simulink model "trifasikos_ask53_trifasikos"  (R2021a)
settings: Solver=ode23tb  StartTime=0.0  StopTime=5.2  MaxStep=1e-4  RelTol=1e-3
libraries: spsSaturableTransformerLib x6, spsCurrentMeasurementLib x5, spsVoltageMeasurementLib x5, spsNeutralLib x4, spsSeriesRLCBranchLib x4, spsControlledVoltageSourceLib x3, spsRMSLib x3, simulink x1, spsMeanLib x1, spsPower3phInstantaneousLib x1, spsDCVoltageSourceLib x1, spspowerguiLib x1
settings Model: Creator=User  LastModifiedBy=epape
settings SolverCC: AlgebraicLoopSolver=TrustRegion
settings DebuggingCC: SFMachineParentedDataDiag=warning

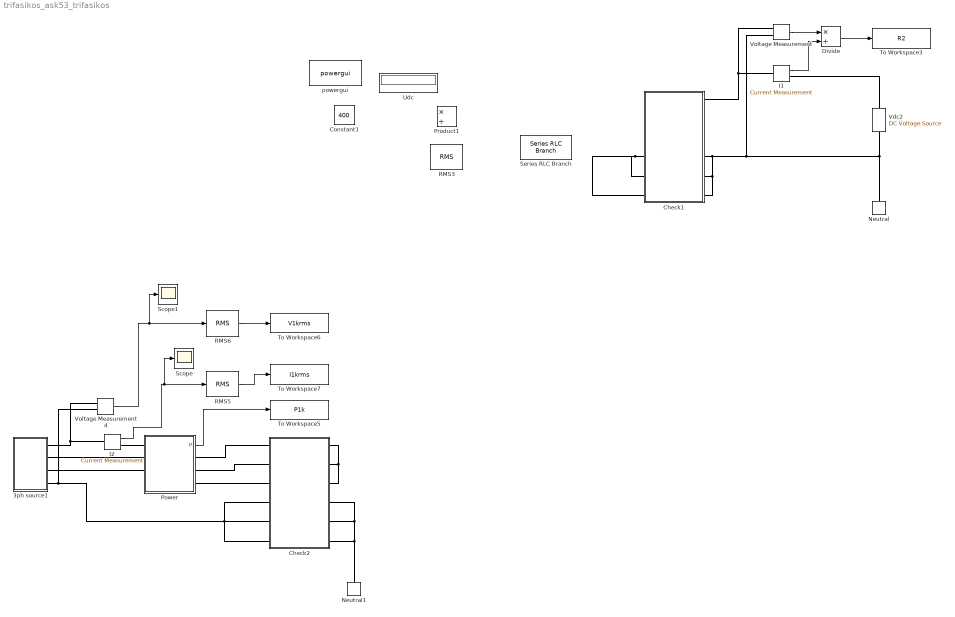
== system trifasikos_ask53_trifasikos ==
  3ph source1 : Subsystem  mask{Vrms=400}
      mask prompts: Vrms "VLL,rms (V)"
  Check1 : Subsystem  mask{PN=12, U1N=230, U2N=115}
      mask prompts: PN "PN (kVA)"; U1N "U1Nph (V)"; U2N "U2Nph (V)"
  Check2 : Subsystem  mask{PN=12, U1N=230, U2N=115}
      mask prompts: PN "PN (kVA)"; U1N "U1Nph (V)"; U2N "U2Nph (V)"
  Constant1 : Constant  Value=400
  Divide : Product  Inputs=*/
  I1 : spsCurrentMeasurementLib/Current Measurement  PhasorSimulation=off  OutputType=Complex  PSBequivalent=0
  I2 : spsCurrentMeasurementLib/Current Measurement  PhasorSimulation=off  OutputType=Complex  PSBequivalent=0
  Neutral : spsNeutralLib/Neutral  LConnTagsString=a  NodeNumber=10
      settings: AttributesFormatString=node %<NodeNumber>  SourceProductBaseCode=PS
  Neutral1 : spsNeutralLib/Neutral  LConnTagsString=a  NodeNumber=10
      settings: AttributesFormatString=node %<NodeNumber>  SourceProductBaseCode=PS
  Power : Subsystem
      mask DialogControl Control2 Prompt: Three phase power measurement
  Product1 : Product  Inputs=*/
  RMS3 : spsRMSLib/RMS  TrueRMS=on  Freq=50  RMSInit=0  Ts=0
  RMS5 : spsRMSLib/RMS  TrueRMS=on  Freq=50  RMSInit=0  Ts=0
  RMS6 : spsRMSLib/RMS  TrueRMS=on  Freq=50  RMSInit=0  Ts=0
  Scope : Scope
  Scope1 : Scope
  Series RLC Branch : spsSeriesRLCBranchLib/Series RLC Branch  LConnTagsString=__new0  RConnTagsString=__new0  BranchType=RLC  Resistance=1  Inductance=1e-3  SetiL0=off  InitialCurrent=0  Capacitance=1e-6  Setx0=off  InitialVoltage=0  Measurements=None
  To Workspace3 : ToWorkspace  VariableName=R2  SaveFormat=Timeseries  SampleTime=-1
  To Workspace5 : ToWorkspace  VariableName=P1k  SaveFormat=Timeseries  SampleTime=-1
  To Workspace6 : ToWorkspace  VariableName=V1krms  SaveFormat=Timeseries  SampleTime=-1
  To Workspace7 : ToWorkspace  VariableName=I1krms  SaveFormat=Timeseries  SampleTime=-1
  Udc : Display
  Vdc2 : spsDCVoltageSourceLib/DC Voltage Source  Amplitude=10  Measurements=None
  Voltage Measurement : spsVoltageMeasurementLib/Voltage Measurement  PhasorSimulation=off  OutputType=Complex  PSBequivalent=0
  Voltage Measurement4 : spsVoltageMeasurementLib/Voltage Measurement  PhasorSimulation=off  OutputType=Complex  PSBequivalent=0
  powergui : spspowerguiLib/powergui  Priority=1  SimulationMode=Continuous  SampleTime=50e-6  frequency=60  Iterations=50  frequencyindice=50  Pbase=100e6  ErrMax=1e-4  UnitsV=kV  UnitsW=MW  buscounter=0  FunctionMessages=off  echomessages=off  EnableUseOfTLC=off  CurrentSourceSwitches=off  DisableSnubberDevices=off  DisableRonSwitches=off  DisableVfSwitches=off  DisplayEquations=off  AutomaticDiscreteSolvers=off  SolverType=Tustin/Backward Euler (TBE)  Interpol=off  ExternalGateDelay=off  methode=off  Ts=100  x0status=blocks  SPID=on  SwTol=0  HookPort=off  NonlinearTolerance=1e-4  nMaxIteration=100  ContinueOnMaxIteration=off  RestoreLinks=warning  ResistiveCurrentMeasurement=off  Frange=[0:2:500]  Ylog=off  Xlog=on  ShowGrid=off  save=off  variable=ZData  structure=0  ZoomFFT=off  StartTime=0.0  cycles=1  DisplayStyle=1  fundamental=60  FreqAxis=off  MaxFrequency=1000  frequencyindicesteady=1  RmsSteady=1  display=off
  wires:
  Divide/1 -> To Workspace3/1
  Voltage Measurement/1 -> Divide/1
  I1/1 -> Divide/2
  Power/1(P) -> To Workspace5/1
  RMS6/1 -> To Workspace6/1
  RMS5/1 -> To Workspace7/1
  Voltage Measurement4/1 -> Scope1/1, RMS6/1
  I2/1 -> Scope/1, RMS5/1
  connections:
  Check1/LConn4 -- Check1/LConn6 -- Check1/LConn5
  3ph source1/RConn4 -- Check2/LConn4 -- Check2/LConn6 -- Check2/LConn5 -- Voltage Measurement4/LConn2
  Neutral1/LConn1 -- Check2/RConn6 -- Check2/RConn4 -- Check2/RConn5
  Check1/RConn4 -- Voltage Measurement/LConn2 -- Neutral/LConn1 -- Vdc2/LConn1 -- Check1/RConn6 -- Check1/RConn5
  I1/LConn1 -- Check1/RConn1 -- Voltage Measurement/LConn1
  I1/RConn1 -- Vdc2/RConn1
  Power/RConn1 -- Check2/LConn1
  Power/RConn2 -- Check2/LConn2
  Power/RConn3 -- Check2/LConn3
  Voltage Measurement4/LConn1 -- 3ph source1/RConn1 -- I2/LConn1
  Power/LConn2 -- 3ph source1/RConn2
  Power/LConn3 -- 3ph source1/RConn3
  Power/LConn1 -- I2/RConn1
  Check2/RConn1 -- Check2/RConn3 -- Check2/RConn2

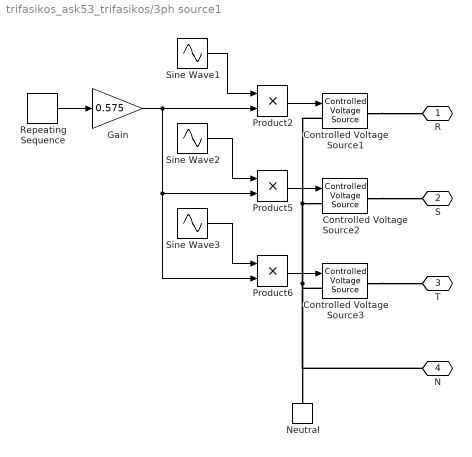
== system trifasikos_ask53_trifasikos/3ph source1 ==
  Controlled Voltage Source1 : spsControlledVoltageSourceLib/Controlled Voltage Source  Initialize=on  Source_Type=AC  Amplitude=0  Phase=0  Frequency=50  Measurements=Voltage
  Controlled Voltage Source2 : spsControlledVoltageSourceLib/Controlled Voltage Source  Initialize=on  Source_Type=AC  Amplitude=0  Phase=0  Frequency=50  Measurements=Voltage
  Controlled Voltage Source3 : spsControlledVoltageSourceLib/Controlled Voltage Source  Initialize=on  Source_Type=AC  Amplitude=0  Phase=0  Frequency=50  Measurements=Voltage
  Gain : Gain  Gain=0.575
  Neutral : spsNeutralLib/Neutral  LConnTagsString=a  NodeNumber=10
      settings: AttributesFormatString=node %<NodeNumber>  SourceProductBaseCode=PS
  Product2 : Product
  Product5 : Product
  Product6 : Product
  Repeating Sequence : simulink/Sources/Repeating Sequence  rep_seq_t=t  rep_seq_y=Vs
  Sine Wave1 : Sin  Amplitude=sqrt(2)  Frequency=100*pi  SampleTime=0
  Sine Wave2 : Sin  Amplitude=sqrt(2)  Frequency=100*pi  Phase=-2*pi/3  SampleTime=0
  Sine Wave3 : Sin  Amplitude=sqrt(2)  Frequency=100*pi  Phase=2*pi/3  SampleTime=0
  R : PMIOPort  Side=Right
  S : PMIOPort  Port=2  Side=Right
  T : PMIOPort  Port=3  Side=Right
  N : PMIOPort  Port=4  Side=Right
  wires:
  Repeating Sequence/1 -> Gain/1
  Product5/1 -> Controlled Voltage Source2/1
  Sine Wave2/1 -> Product5/1
  Product6/1 -> Controlled Voltage Source3/1
  Sine Wave3/1 -> Product6/1
  Product2/1 -> Controlled Voltage Source1/1
  Sine Wave1/1 -> Product2/1
  Gain/1 -> Product6/2, Product5/2, Product2/2
  connections:
  Controlled Voltage Source2/RConn1 -- S/RConn1
  Controlled Voltage Source1/LConn1 -- Controlled Voltage Source2/LConn1 -- Controlled Voltage Source3/LConn1 -- N/RConn1 -- Neutral/LConn1
  Controlled Voltage Source3/RConn1 -- T/RConn1
  Controlled Voltage Source1/RConn1 -- R/RConn1

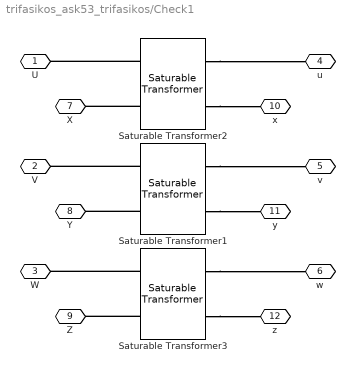
== system trifasikos_ask53_trifasikos/Check1 ==
  Saturable Transformer1 : spsSaturableTransformerLib/Saturable Transformer  ThreeWindings=off  Hysteresis=off  DataFile='hysteresis.mat'  Measurements=None  UNITS=pu  NominalPower=[4e3 50]  Winding1=[230 0.022273 0.015903]  Winding2=[122 0.024298 0.019083]  Winding3=[3.15e+05 0.00245 0.098001]  Saturation=[0 0;0.031714 0.76205;0.037813 0.86926;0.045538 0.94653;0.060175 1.0141;0.080911 1.0624;0.14637 1.159]  CoreLoss=35.539  BreakLoop=off  DiscreteSolver=Trapezoidal iterative  DataType=off  InitialFlux=0  TransfoNumber=1
      settings: SourceProductBaseCode=PS
  Saturable Transformer2 : spsSaturableTransformerLib/Saturable Transformer  ThreeWindings=off  Hysteresis=off  DataFile='hysteresis.mat'  Measurements=None  UNITS=SI  NominalPower=[4e3 50]  Winding1=[230 0.29456 0.00066946]  Winding2=[122 0.090413 0.00022602]  Winding3=[3.15e+05 60775 7738.2]  Saturation=[0 0;0.78001 0.789;0.93001 0.9;1.12 0.98;1.48 1.05;1.99 1.1;3.6 1.2]  CoreLoss=470  BreakLoop=off  DiscreteSolver=Trapezoidal iterative  DataType=on  InitialFlux=0  TransfoNumber=1
      settings: SourceProductBaseCode=PS
  Saturable Transformer3 : spsSaturableTransformerLib/Saturable Transformer  ThreeWindings=off  Hysteresis=off  DataFile='hysteresis.mat'  Measurements=None  UNITS=pu  NominalPower=[4e3 50]  Winding1=[230 0.022273 0.015903]  Winding2=[122 0.024298 0.019083]  Winding3=[3.15e+05 0.00245 0.098001]  Saturation=[0 0;0.031714 0.76205;0.037813 0.86926;0.045538 0.94653;0.060175 1.0141;0.080911 1.0624;0.14637 1.159]  CoreLoss=35.539  BreakLoop=off  DiscreteSolver=Trapezoidal iterative  DataType=off  InitialFlux=0  TransfoNumber=1
      settings: SourceProductBaseCode=PS
  U : PMIOPort  Side=Left
  V : PMIOPort  Port=2  Side=Left
  W : PMIOPort  Port=3  Side=Left
  u : PMIOPort  Port=4  Side=Right
  v : PMIOPort  Port=5  Side=Right
  w : PMIOPort  Port=6  Side=Right
  X : PMIOPort  Port=7  Side=Left
  Y : PMIOPort  Port=8  Side=Left
  Z : PMIOPort  Port=9  Side=Left
  x : PMIOPort  Port=10  Side=Right
  y : PMIOPort  Port=11  Side=Right
  z : PMIOPort  Port=12  Side=Right
  connections:
  Saturable Transformer1/LConn2 -- Y/RConn1
  Saturable Transformer2/LConn1 -- U/RConn1
  Saturable Transformer1/LConn1 -- V/RConn1
  Saturable Transformer3/LConn1 -- W/RConn1
  Saturable Transformer2/LConn2 -- X/RConn1
  Saturable Transformer3/LConn2 -- Z/RConn1
  Saturable Transformer2/RConn1 -- u/RConn1
  Saturable Transformer2/RConn2 -- x/RConn1
  Saturable Transformer1/RConn1 -- v/RConn1
  Saturable Transformer1/RConn2 -- y/RConn1
  Saturable Transformer3/RConn1 -- w/RConn1
  Saturable Transformer3/RConn2 -- z/RConn1

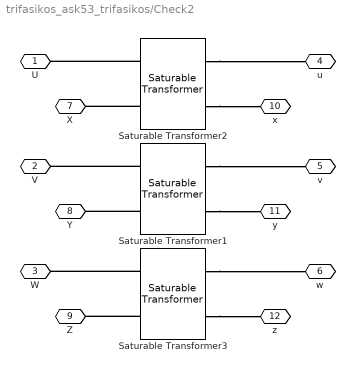
== system trifasikos_ask53_trifasikos/Check2 ==
  Saturable Transformer1 : spsSaturableTransformerLib/Saturable Transformer  ThreeWindings=off  Hysteresis=off  DataFile='hysteresis.mat'  Measurements=None  UNITS=pu  NominalPower=[4e3 50]  Winding1=[230 0.022273 0.015903]  Winding2=[122 0.024298 0.019083]  Winding3=[3.15e+05 0.00245 0.098001]  Saturation=[0 0;0.031714 0.76205;0.037813 0.86926;0.045538 0.94653;0.060175 1.0141;0.080911 1.0624;0.14637 1.159]  CoreLoss=35.539  BreakLoop=off  DiscreteSolver=Trapezoidal iterative  DataType=off  InitialFlux=0  TransfoNumber=1
      settings: SourceProductBaseCode=PS
  Saturable Transformer2 : spsSaturableTransformerLib/Saturable Transformer  ThreeWindings=off  Hysteresis=off  DataFile='hysteresis.mat'  Measurements=None  UNITS=SI  NominalPower=[4e3 50]  Winding1=[230 0.29456 0.00066946]  Winding2=[122 0.090413 0.00022602]  Winding3=[3.15e+05 60775 7738.2]  Saturation=[0 0;0.78001 0.789;0.93001 0.9;1.12 0.98;1.48 1.05;1.99 1.1;3.6 1.2]  CoreLoss=470  BreakLoop=off  DiscreteSolver=Trapezoidal iterative  DataType=on  InitialFlux=0  TransfoNumber=1
      settings: SourceProductBaseCode=PS
  Saturable Transformer3 : spsSaturableTransformerLib/Saturable Transformer  ThreeWindings=off  Hysteresis=off  DataFile='hysteresis.mat'  Measurements=None  UNITS=pu  NominalPower=[4e3 50]  Winding1=[230 0.022273 0.015903]  Winding2=[122 0.024298 0.019083]  Winding3=[3.15e+05 0.00245 0.098001]  Saturation=[0 0;0.031714 0.76205;0.037813 0.86926;0.045538 0.94653;0.060175 1.0141;0.080911 1.0624;0.14637 1.159]  CoreLoss=35.539  BreakLoop=off  DiscreteSolver=Trapezoidal iterative  DataType=off  InitialFlux=0  TransfoNumber=1
      settings: SourceProductBaseCode=PS
  U : PMIOPort  Side=Left
  V : PMIOPort  Port=2  Side=Left
  W : PMIOPort  Port=3  Side=Left
  u : PMIOPort  Port=4  Side=Right
  v : PMIOPort  Port=5  Side=Right
  w : PMIOPort  Port=6  Side=Right
  X : PMIOPort  Port=7  Side=Left
  Y : PMIOPort  Port=8  Side=Left
  Z : PMIOPort  Port=9  Side=Left
  x : PMIOPort  Port=10  Side=Right
  y : PMIOPort  Port=11  Side=Right
  z : PMIOPort  Port=12  Side=Right
  connections:
  Saturable Transformer1/LConn2 -- Y/RConn1
  Saturable Transformer2/LConn1 -- U/RConn1
  Saturable Transformer1/LConn1 -- V/RConn1
  Saturable Transformer3/LConn1 -- W/RConn1
  Saturable Transformer2/LConn2 -- X/RConn1
  Saturable Transformer3/LConn2 -- Z/RConn1
  Saturable Transformer2/RConn1 -- u/RConn1
  Saturable Transformer2/RConn2 -- x/RConn1
  Saturable Transformer1/RConn1 -- v/RConn1
  Saturable Transformer1/RConn2 -- y/RConn1
  Saturable Transformer3/RConn1 -- w/RConn1
  Saturable Transformer3/RConn2 -- z/RConn1

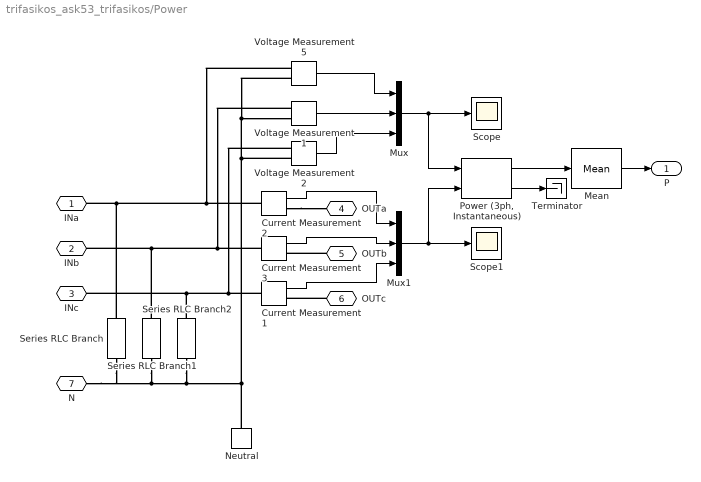
== system trifasikos_ask53_trifasikos/Power ==
  Current Measurement1 : spsCurrentMeasurementLib/Current Measurement  PhasorSimulation=off  OutputType=Complex  PSBequivalent=0
  Current Measurement2 : spsCurrentMeasurementLib/Current Measurement  PhasorSimulation=off  OutputType=Complex  PSBequivalent=0
  Current Measurement3 : spsCurrentMeasurementLib/Current Measurement  PhasorSimulation=off  OutputType=Complex  PSBequivalent=0
  Mean : spsMeanLib/Mean  Freq=50  Vinit=0  Ts=0
  Mux : Mux  Inputs=3
  Mux1 : Mux  Inputs=3
  Neutral : spsNeutralLib/Neutral  LConnTagsString=a  NodeNumber=10
      settings: AttributesFormatString=node %<NodeNumber>  SourceProductBaseCode=PS
  "Power (3ph, Instantaneous)" : spsPower3phInstantaneousLib/Power (3ph, Instantaneous)
  Scope : Scope
  Scope1 : Scope
  Series RLC Branch : spsSeriesRLCBranchLib/Series RLC Branch  LConnTagsString=__new0  RConnTagsString=__new0  BranchType=R  Resistance=1e6  Inductance=1e-3  SetiL0=off  InitialCurrent=0  Capacitance=1e-6  Setx0=off  InitialVoltage=0  Measurements=None
  Series RLC Branch1 : spsSeriesRLCBranchLib/Series RLC Branch  LConnTagsString=__new0  RConnTagsString=__new0  BranchType=R  Resistance=1e6  Inductance=1e-3  SetiL0=off  InitialCurrent=0  Capacitance=1e-6  Setx0=off  InitialVoltage=0  Measurements=None
  Series RLC Branch2 : spsSeriesRLCBranchLib/Series RLC Branch  LConnTagsString=__new0  RConnTagsString=__new0  BranchType=R  Resistance=1e6  Inductance=1e-3  SetiL0=off  InitialCurrent=0  Capacitance=1e-6  Setx0=off  InitialVoltage=0  Measurements=None
  Terminator : Terminator
  Voltage Measurement1 : spsVoltageMeasurementLib/Voltage Measurement  PhasorSimulation=off  OutputType=Complex  PSBequivalent=0
  Voltage Measurement2 : spsVoltageMeasurementLib/Voltage Measurement  PhasorSimulation=off  OutputType=Complex  PSBequivalent=0
  Voltage Measurement5 : spsVoltageMeasurementLib/Voltage Measurement  PhasorSimulation=off  OutputType=Complex  PSBequivalent=0
  INa : PMIOPort  Side=Left
  INb : PMIOPort  Port=2  Side=Left
  INc : PMIOPort  Port=3  Side=Left
  OUTa : PMIOPort  Port=4  Side=Right
  OUTb : PMIOPort  Port=5  Side=Right
  OUTc : PMIOPort  Port=6  Side=Right
  N : PMIOPort  Port=7  Side=Left
  P : Outport
  wires:
  "Power (3ph, Instantaneous)"/1 -> Mean/1
  Mux/1 -> "Power (3ph, Instantaneous)"/1, Scope/1
  Voltage Measurement5/1 -> Mux/1
  Mux1/1 -> "Power (3ph, Instantaneous)"/2, Scope1/1
  Voltage Measurement1/1 -> Mux/2
  Voltage Measurement2/1 -> Mux/3
  Current Measurement3/1 -> Mux1/2
  Current Measurement2/1 -> Mux1/1
  Current Measurement1/1 -> Mux1/3
  "Power (3ph, Instantaneous)"/2 -> Terminator/1
  Mean/1 -> P/1
  connections:
  Current Measurement1/LConn1 -- Voltage Measurement2/LConn1 -- Series RLC Branch2/LConn1 -- INc/RConn1
  Current Measurement3/LConn1 -- Voltage Measurement1/LConn1 -- Series RLC Branch1/LConn1 -- INb/RConn1
  Current Measurement2/LConn1 -- Voltage Measurement5/LConn1 -- Series RLC Branch/LConn1 -- INa/RConn1
  Voltage Measurement5/LConn2 -- Series RLC Branch/RConn1 -- N/RConn1 -- Series RLC Branch1/RConn1 -- Series RLC Branch2/RConn1 -- Neutral/LConn1 -- Voltage Measurement2/LConn2 -- Voltage Measurement1/LConn2
  Current Measurement2/RConn1 -- OUTa/RConn1
  OUTb/RConn1 -- Current Measurement3/RConn1
  OUTc/RConn1 -- Current Measurement1/RConn1
